simulink model "Dahlin"  (R2023b)
settings: Solver=VariableStepAuto  StartTime=0.0  StopTime=200  RelTol=1e-3
values from neighbouring files (symbols this model uses):
  Tm = 2.5    [Lab3.m]
  Ts = 0.5    [Lab3.m]
undefined symbols (not defined in the file or in its folder): denF, denRbun, denRe, numF, numRbun, numRe
settings Model: Creator=raluc  LastModifiedBy=raluc

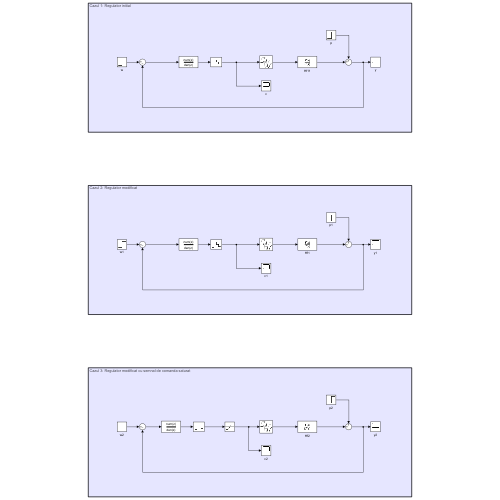
[thumbnail: Simulink's stored preview of the top-level diagram]
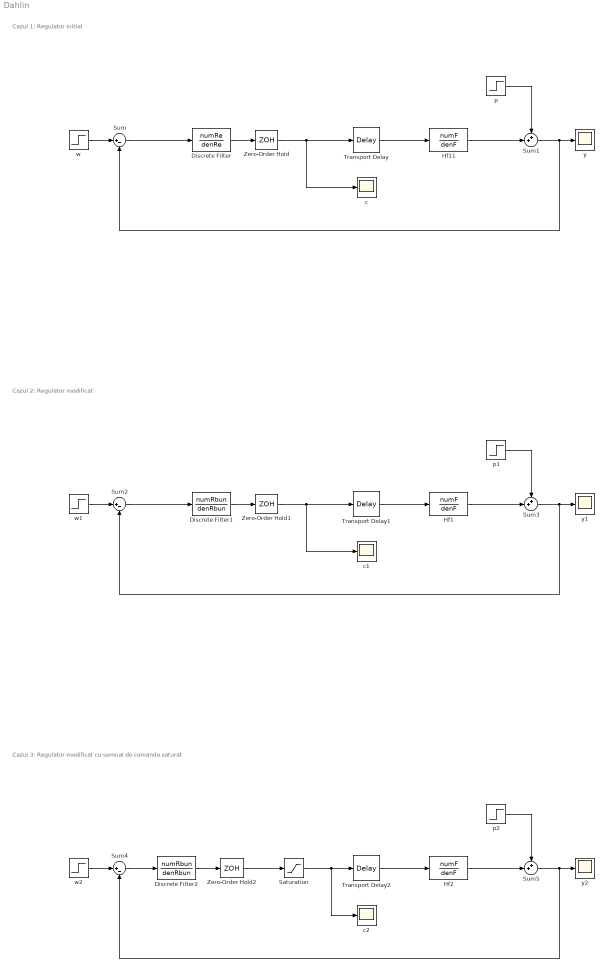
== system Dahlin ==
  note: Cazul 1: Regulator initial
  note: Cazul 2: Regulator modificat
  note: Cazul 3: Regulator modificat cu semnal de comanda saturat
  Discrete Filter : DiscreteFilter  Numerator=numRe  Denominator=denRe
  Discrete Filter1 : DiscreteFilter  Numerator=numRbun  Denominator=denRbun
  Discrete Filter2 : DiscreteFilter  Numerator=numRbun  Denominator=denRbun
  Hf1 : TransferFcn  Numerator=numF  Denominator=denF
  Hf11 : TransferFcn  Numerator=numF  Denominator=denF
  Hf2 : TransferFcn  Numerator=numF  Denominator=denF
  Saturation : Saturate  UpperLimit=1  LowerLimit=0
  Sum : Sum  Inputs=|+-
  Sum1 : Sum  Inputs=++|
  Sum2 : Sum  Inputs=|+-
  Sum3 : Sum  Inputs=++|
  Sum4 : Sum  Inputs=|+-
  Sum5 : Sum  Inputs=++|
  Transport Delay : TransportDelay  DelayTime=Tm
  Transport Delay1 : TransportDelay  DelayTime=Tm
  Transport Delay2 : TransportDelay  DelayTime=Tm
  Zero-Order Hold : ZeroOrderHold  SampleTime=Ts
  Zero-Order Hold1 : ZeroOrderHold  SampleTime=Ts
  Zero-Order Hold2 : ZeroOrderHold  SampleTime=Ts
  c : Scope
  c1 : Scope
  c2 : Scope
  p : Step  After=0  SampleTime=0
  p1 : Step  After=0  SampleTime=0
  p2 : Step  After=0  SampleTime=0
  w : Step  SampleTime=0
  w1 : Step  SampleTime=0
  w2 : Step  SampleTime=0
  y : Scope
  y1 : Scope
  y2 : Scope
  wires:
  w/1 -> Sum/1
  Sum/1 -> Discrete Filter/1
  Transport Delay/1 -> Hf11/1
  Sum1/1 -> Sum/2, y/1
  Hf11/1 -> Sum1/2
  p/1 -> Sum1/1
  Discrete Filter/1 -> Zero-Order Hold/1
  Zero-Order Hold/1 -> c/1, Transport Delay/1
  w1/1 -> Sum2/1
  Discrete Filter1/1 -> Zero-Order Hold1/1
  p1/1 -> Sum3/1
  Hf1/1 -> Sum3/2
  Sum3/1 -> Sum2/2, y1/1
  Zero-Order Hold1/1 -> c1/1, Transport Delay1/1
  Sum2/1 -> Discrete Filter1/1
  Transport Delay1/1 -> Hf1/1
  p2/1 -> Sum5/1
  Discrete Filter2/1 -> Zero-Order Hold2/1
  w2/1 -> Sum4/1
  Transport Delay2/1 -> Hf2/1
  Sum5/1 -> Sum4/2, y2/1
  Sum4/1 -> Discrete Filter2/1
  Hf2/1 -> Sum5/2
  Zero-Order Hold2/1 -> Saturation/1
  Saturation/1 -> c2/1, Transport Delay2/1
